simulink model "SiEngine"  (R2020a)
settings: Solver=VariableStepAuto  StartTime=0.0  StopTime=inf  RelTol=1e-3  EnableMultiTasking=on
model workspace (MAT data in the model file):
  AccPwrbp = [0 1.5]
  AccSpdbp = [300 750]
  AfrStoich = 14.6
  TimeCnstECP = 0.125
  TimeCnstEGR = 0.125
  TimeCnstETC = 0.085
  TimeCnstICP = 0.125
  TimeCnstIVL = 0.125
  TimeCnstSWVA = 0.125
  TimeCnstVCR = 0.125
  TimeCnstVGT = 0.15
  TimeCnstVIRL = 0.125
  TimeCnstWGA = 0.15
  f_twc_eff_co = [0.17 0.25 0.45 0.99 0.99 0.99 0.99]
  f_twc_eff_hc = [0.21 0.375 0.75 0.98 0.98 0.98 0.98]
  f_twc_eff_lam = [0.909090909 0.944055944 0.979020979 1 1.013986014 1.048951049 1.083916084]
  f_twc_eff_nox = [0.98 0.98 0.98 0.97 0.05 0.02 0]
libraries: autolibpowerinfoutils x1, autolibutils x1
settings Model: ModifiedByFormat=The MathWorks, Inc.  OrderedModelArguments=off  Creator=The MathWorks, Inc.  LastModifiedBy=The MathWorks, Inc.
settings SolverCC: DecoupledContinuousIntegration=on
settings DataIOCC: DSMLogging=off  ReturnWorkspaceOutputs=off
settings DebuggingCC: ModelReferenceExtraNoncontSigs=none  ArithmeticOperatorsInVariantConditions=warning
settings SFSimCC: SimUseLocalCustomCode=off  CustomCodeUndefinedFunction=UseInterfaceOnly
settings RTWCC: RTWUseLocalCustomCode=off
settings CodeAppCC: StateflowObjectComments=on
settings GRTTargetCC: TargetLangStandard=C89/C90 (ANSI)
settings ConfigComp: CovMetricSettings=dsw  CovHtmlReporting=on  CovSaveCumulativeToWorkspaceVar=on  CovSaveSingleToWorkspaceVar=on  CovShowResultsExplorer=off  CovExternalEMLEnable=off
settings SimscapeCC: SimscapeNormalizeSystem=off  SimscapeNominalValues={1, 'bar'; 1, 'cm^3/s'; 1, 'bar*kg/s'; 1, 'kJ/kg'; 1, 'kW'; };

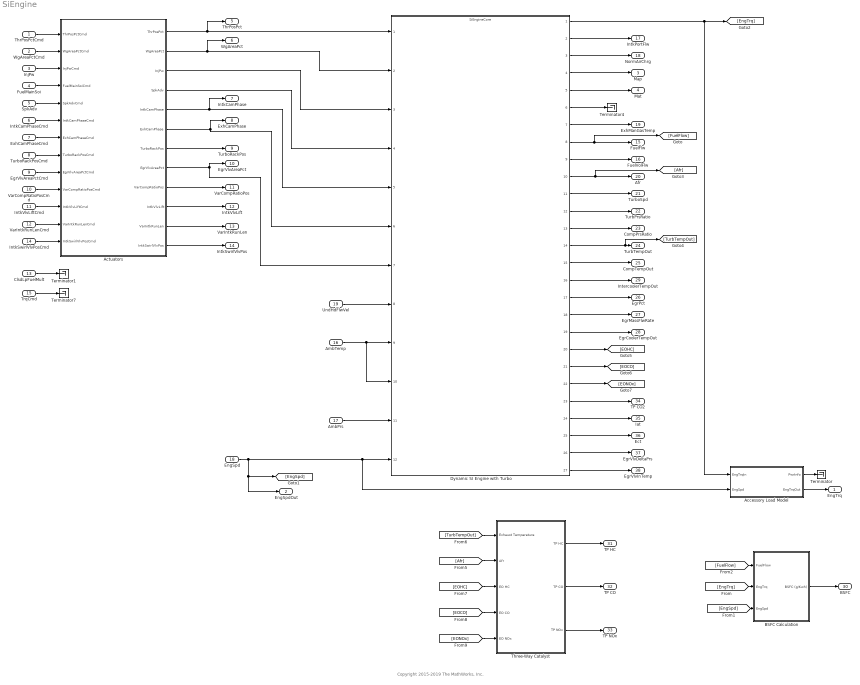
== system SiEngine ==
  note: Copyright 2015-2019 The MathWorks, Inc.
  ThrPosPctCmd : Inport
  WgAreaPctCmd : Inport  Port=2
  InjPw : Inport  Port=3
  FuelMainSoi : Inport  Port=4
  SpkAdv : Inport  Port=5
  IntkCamPhaseCmd : Inport  Port=6
  ExhCamPhaseCmd : Inport  Port=7
  TurboRackPosCmd : Inport  Port=8
  EgrVlvAreaPctCmd : Inport  Port=9
  VarCompRatioPosCmd : Inport  Port=10
  IntkVlvLiftCmd : Inport  Port=11
  VarIntkRunLenCmd : Inport  Port=12
  ClsdLpFuelMult : Inport  Port=13  Unit=1
  IntkSwirlVlvPosCmd : Inport  Port=14
  TrqCmd : Inport  Port=15  Unit=N*m
  AmbTemp : Inport  Port=16
  AmbPrs : Inport  Port=17
  EngSpd : Inport  Port=18  Interpolate=off
  UndHdFlwVel : Inport  Port=19
  Accessory Load Model : Subsystem
  Actuators : Subsystem
  BSFC Calculation : Subsystem
  Dynamic SI Engine with Turbo : ModelReference  ModelNameDialog=SiEngineCore.slx  SimulationMode=Normal  ModelReferenceVersion=1.557
  Terminator{,1,4,7} (4 alike) : Terminator
  Three-Way Catalyst : Subsystem
  EngTrq : Outport  Unit=N*m  VectorParamsAs1DForOutWhenUnconnected=off
  EngSpdOut : Outport  Port=2  VectorParamsAs1DForOutWhenUnconnected=off
  Map : Outport  Port=3  VectorParamsAs1DForOutWhenUnconnected=off
  Mat : Outport  Port=4  VectorParamsAs1DForOutWhenUnconnected=off
  ThrPosPct : Outport  Port=5  VectorParamsAs1DForOutWhenUnconnected=off
  WgAreaPct : Outport  Port=6  VectorParamsAs1DForOutWhenUnconnected=off
  IntkCamPhase : Outport  Port=7  VectorParamsAs1DForOutWhenUnconnected=off
  ExhCamPhase : Outport  Port=8  VectorParamsAs1DForOutWhenUnconnected=off
  TurboRackPos : Outport  Port=9  VectorParamsAs1DForOutWhenUnconnected=off
  EgrVlvAreaPct : Outport  Port=10  VectorParamsAs1DForOutWhenUnconnected=off
  VarCompRatioPos : Outport  Port=11  VectorParamsAs1DForOutWhenUnconnected=off
  IntkVlvLift : Outport  Port=12  VectorParamsAs1DForOutWhenUnconnected=off
  VarIntkRunLen : Outport  Port=13  VectorParamsAs1DForOutWhenUnconnected=off
  IntkSwirlVlvPos : Outport  Port=14  VectorParamsAs1DForOutWhenUnconnected=off
  FuelFlw : Outport  Port=15  VectorParamsAs1DForOutWhenUnconnected=off
  FuelVolFlw : Outport  Port=16  VectorParamsAs1DForOutWhenUnconnected=off
  IntkPortFlw : Outport  Port=17  VectorParamsAs1DForOutWhenUnconnected=off
  NormAirChrg : Outport  Port=18  VectorParamsAs1DForOutWhenUnconnected=off
  ExhManGasTemp : Outport  Port=19  VectorParamsAs1DForOutWhenUnconnected=off
  Afr : Outport  Port=20  VectorParamsAs1DForOutWhenUnconnected=off
  TurboSpd : Outport  Port=21  VectorParamsAs1DForOutWhenUnconnected=off
  TurbPrsRatio : Outport  Port=22  VectorParamsAs1DForOutWhenUnconnected=off
  CompPrsRatio : Outport  Port=23  VectorParamsAs1DForOutWhenUnconnected=off
  TurbTempOut : Outport  Port=24  VectorParamsAs1DForOutWhenUnconnected=off
  CompTempOut : Outport  Port=25  VectorParamsAs1DForOutWhenUnconnected=off
  EgrPct : Outport  Port=26  Unit=%  VectorParamsAs1DForOutWhenUnconnected=off
  EgrMassFlwRate : Outport  Port=27  Unit=kg/s  VectorParamsAs1DForOutWhenUnconnected=off
  EgrCoolerTempOut : Outport  Port=28  Unit=K  VectorParamsAs1DForOutWhenUnconnected=off
  IntercoolerTempOut : Outport  Port=29  VectorParamsAs1DForOutWhenUnconnected=off
  BSFC : Outport  Port=30  Unit=g/(kW*hr)  VectorParamsAs1DForOutWhenUnconnected=off
  TP HC : Outport  Port=31  VectorParamsAs1DForOutWhenUnconnected=off
  TP CO : Outport  Port=32  VectorParamsAs1DForOutWhenUnconnected=off
  TP NOx : Outport  Port=33  VectorParamsAs1DForOutWhenUnconnected=off
  TP CO2 : Outport  Port=34  VectorParamsAs1DForOutWhenUnconnected=off
  Iat : Outport  Port=35  VectorParamsAs1DForOutWhenUnconnected=off
  Ect : Outport  Port=36  VectorParamsAs1DForOutWhenUnconnected=off
  EgrVlvDeltaPrs : Outport  Port=37  VectorParamsAs1DForOutWhenUnconnected=off
  EgrVlvInTemp : Outport  Port=38  VectorParamsAs1DForOutWhenUnconnected=off
  wires:
  Dynamic SI Engine with Turbo/2 -> IntkPortFlw/1
  Dynamic SI Engine with Turbo/6 -> Terminator4/1
  Dynamic SI Engine with Turbo/7 -> ExhManGasTemp/1
  Dynamic SI Engine with Turbo/4 -> Map/1
  Dynamic SI Engine with Turbo/5 -> Mat/1
  SpkAdv/1 -> Actuators/5(SpkAdvCmd)
  InjPw/1 -> Actuators/3(InjPwCmd)
  EngSpd/1 -> EngSpdOut/1, [EngSpd], Dynamic SI Engine with Turbo/12, Accessory Load Model/2(EngSpd)
  [FuelFlow] -> BSFC Calculation/1(FuelFlow)
  [EngTrq] -> BSFC Calculation/2(EngTrq)
  [EngSpd] -> BSFC Calculation/3(EngSpd)
  BSFC Calculation/1(BSFC (g/Kwh)) -> BSFC/1
  Dynamic SI Engine with Turbo/1 -> Accessory Load Model/1(EngTrqIn), [EngTrq]
  Three-Way Catalyst/1(TP HC) -> TP HC/1
  Three-Way Catalyst/2(TP CO) -> TP CO/1
  Three-Way Catalyst/3(TP NOx) -> TP NOx/1
  [TurbTempOut] -> Three-Way Catalyst/1(Exhaust Temperature)
  [Afr] -> Three-Way Catalyst/2(Afr)
  ThrPosPctCmd/1 -> Actuators/1(ThrPosPctCmd)
  WgAreaPctCmd/1 -> Actuators/2(WgAreaPctCmd)
  IntkCamPhaseCmd/1 -> Actuators/6(IntkCamPhaseCmd)
  ExhCamPhaseCmd/1 -> Actuators/7(ExhCamPhaseCmd)
  Dynamic SI Engine with Turbo/8 -> [FuelFlow], FuelFlw/1
  Dynamic SI Engine with Turbo/10 -> [Afr], Afr/1
  TrqCmd/1 -> Terminator7/1
  Dynamic SI Engine with Turbo/3 -> NormAirChrg/1
  Dynamic SI Engine with Turbo/14 -> TurbTempOut/1, [TurbTempOut]
  [EOHC] -> Three-Way Catalyst/3(EO HC)
  [EOCO] -> Three-Way Catalyst/4(EO CO)
  [EONOx] -> Three-Way Catalyst/5(EO NOx)
  UndHdFlwVel/1 -> Dynamic SI Engine with Turbo/8
  AmbTemp/1 -> Dynamic SI Engine with Turbo/10, Dynamic SI Engine with Turbo/9
  AmbPrs/1 -> Dynamic SI Engine with Turbo/11
  Actuators/1(ThrPosPct) -> Dynamic SI Engine with Turbo/1, ThrPosPct/1
  Actuators/2(WgAreaPct) -> Dynamic SI Engine with Turbo/2, WgAreaPct/1
  Actuators/3(InjPw) -> Dynamic SI Engine with Turbo/3
  Actuators/4(SpkAdv) -> Dynamic SI Engine with Turbo/4
  Actuators/5(IntkCamPhase) -> Dynamic SI Engine with Turbo/5, IntkCamPhase/1
  Actuators/6(ExhCamPhase) -> Dynamic SI Engine with Turbo/6, ExhCamPhase/1
  FuelMainSoi/1 -> Actuators/4(FuelMainSoiCmd)
  TurboRackPosCmd/1 -> Actuators/8(TurboRackPosCmd)
  EgrVlvAreaPctCmd/1 -> Actuators/9(EgrVlvAreaPctCmd)
  VarCompRatioPosCmd/1 -> Actuators/10(VarCompRatioPosCmd)
  IntkVlvLiftCmd/1 -> Actuators/11(IntkVlvLiftCmd)
  VarIntkRunLenCmd/1 -> Actuators/12(VarIntkRunLenCmd)
  IntkSwirlVlvPosCmd/1 -> Actuators/13(IntkSwirlVlvPosCmd)
  Actuators/7(TurboRackPos) -> TurboRackPos/1
  Actuators/8(EgrVlvAreaPct) -> Dynamic SI Engine with Turbo/7, EgrVlvAreaPct/1
  Actuators/9(VarCompRatioPos) -> VarCompRatioPos/1
  Actuators/10(IntkVlvLift) -> IntkVlvLift/1
  Actuators/11(VarIntkRunLen) -> VarIntkRunLen/1
  Actuators/12(IntkSwirlVlvPos) -> IntkSwirlVlvPos/1
  Dynamic SI Engine with Turbo/15 -> CompTempOut/1
  Dynamic SI Engine with Turbo/16 -> IntercoolerTempOut/1
  Dynamic SI Engine with Turbo/13 -> CompPrsRatio/1
  Dynamic SI Engine with Turbo/12 -> TurbPrsRatio/1
  Dynamic SI Engine with Turbo/11 -> TurboSpd/1
  Dynamic SI Engine with Turbo/23 -> TP CO2/1
  Dynamic SI Engine with Turbo/22 -> [EONOx]
  Dynamic SI Engine with Turbo/21 -> [EOCO]
  Dynamic SI Engine with Turbo/20 -> [EOHC]
  Dynamic SI Engine with Turbo/17 -> EgrPct/1
  Dynamic SI Engine with Turbo/18 -> EgrMassFlwRate/1
  Dynamic SI Engine with Turbo/19 -> EgrCoolerTempOut/1
  Dynamic SI Engine with Turbo/25 -> Ect/1
  Dynamic SI Engine with Turbo/26 -> EgrVlvDeltaPrs/1
  Dynamic SI Engine with Turbo/27 -> EgrVlvInTemp/1
  Dynamic SI Engine with Turbo/24 -> Iat/1
  Accessory Load Model/2(EngTrqOut) -> EngTrq/1
  Accessory Load Model/1(PwrInfo) -> Terminator/1
  Dynamic SI Engine with Turbo/9 -> FuelVolFlw/1
  ClsdLpFuelMult/1 -> Terminator1/1

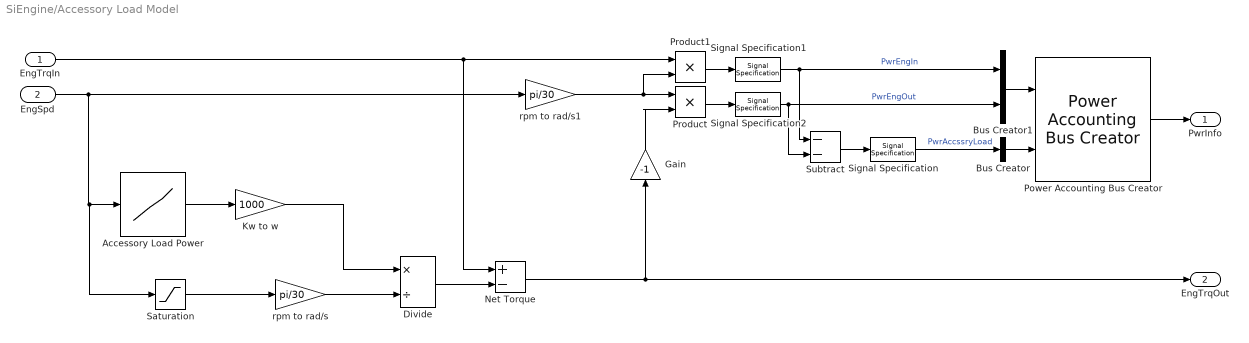
== system SiEngine/Accessory Load Model ==
  EngTrqIn : Inport
  EngSpd : Inport  Port=2
  Accessory Load Power : Lookup_n-D  NumberOfTableDimensions=1  LookupTableObject=''  BreakpointsForDimension1=AccSpdbp  Table=AccPwrbp  ExtrapMethod=Clip  InternalRulePriority=Speed  RndMeth=Simplest  InputSameDT=on
  Bus Creator : BusCreator  Inputs=1
  Bus Creator1 : BusCreator  Inputs=2
  Divide : Product  Inputs=*/
  Gain : Gain  Gain=-1
  Kw to w : Gain  Gain=1000
  Net Torque : Sum  Inputs=+-
  Power Accounting Bus Creator : autolibpowerinfoutils/Power Accounting Bus Creator  AssctBlkSelPopup=Parent  RefBlkName='libraryname/blkname'  PwrTrnsfrdCheckBox=on  PwrNotTrnsfrdCheckBox=on  PwrStoredCheckBox=off  aMode=aMode
      settings: SourceProductBaseCode=PW,MT,VE,VP
  Product : Product
  Product1 : Product
  Saturation : Saturate  UpperLimit=Inf  LowerLimit=300
  Signal Specification : SignalSpecification  Unit=W
  Signal Specification1 : SignalSpecification  Unit=W
  Signal Specification2 : SignalSpecification  Unit=W
  Subtract : Sum  Inputs=--
  rpm to rad/s : Gain  Gain=pi/30
  rpm to rad/s1 : Gain  Gain=pi/30
  PwrInfo : Outport  VectorParamsAs1DForOutWhenUnconnected=off
  EngTrqOut : Outport  Port=2  Unit=N*m  VectorParamsAs1DForOutWhenUnconnected=off
  wires:
  Divide/1 -> Net Torque/2
  Accessory Load Power/1 -> Kw to w/1
  EngSpd/1 -> Saturation/1, Accessory Load Power/1, rpm to rad/s1/1
  Saturation/1 -> rpm to rad/s/1
  rpm to rad/s/1 -> Divide/2
  Net Torque/1 -> EngTrqOut/1, Gain/1
  Bus Creator/1 -> Power Accounting Bus Creator/2
  Kw to w/1 -> Divide/1
  Bus Creator1/1 -> Power Accounting Bus Creator/1
  EngTrqIn/1 -> Product1/1, Net Torque/1
  Subtract/1 -> Signal Specification/1
  Signal Specification/1 -> Bus Creator/1  "PwrAccssryLoad"
  Power Accounting Bus Creator/1 -> PwrInfo/1
  Product/1 -> Signal Specification2/1
  Product1/1 -> Signal Specification1/1
  rpm to rad/s1/1 -> Product1/2, Product/1
  Signal Specification1/1 -> Subtract/1, Bus Creator1/1  "PwrEngIn"
  Signal Specification2/1 -> Subtract/2, Bus Creator1/2  "PwrEngOut"
  Gain/1 -> Product/2

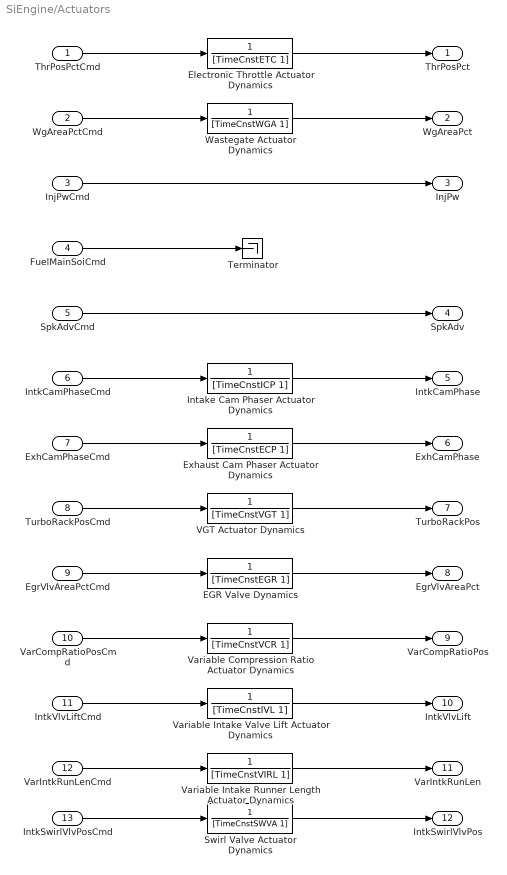
== system SiEngine/Actuators ==
  ThrPosPctCmd : Inport  Unit=%
  WgAreaPctCmd : Inport  Port=2  Unit=%
  InjPwCmd : Inport  Port=3  Unit=ms
  FuelMainSoiCmd : Inport  Port=4  Unit=deg
  SpkAdvCmd : Inport  Port=5  Unit=deg
  IntkCamPhaseCmd : Inport  Port=6  Unit=deg
  ExhCamPhaseCmd : Inport  Port=7  Unit=deg
  TurboRackPosCmd : Inport  Port=8  Unit=1
  EgrVlvAreaPctCmd : Inport  Port=9  Unit=%
  VarCompRatioPosCmd : Inport  Port=10
  IntkVlvLiftCmd : Inport  Port=11
  VarIntkRunLenCmd : Inport  Port=12
  IntkSwirlVlvPosCmd : Inport  Port=13
  EGR Valve Dynamics : TransferFcn  Denominator=[TimeCnstEGR 1]
  Electronic Throttle Actuator Dynamics : TransferFcn  Denominator=[TimeCnstETC 1]
  Exhaust Cam Phaser Actuator Dynamics : TransferFcn  Denominator=[TimeCnstECP 1]
  Intake Cam Phaser Actuator Dynamics : TransferFcn  Denominator=[TimeCnstICP 1]
  Swirl Valve Actuator Dynamics : TransferFcn  Denominator=[TimeCnstSWVA 1]
  Terminator : Terminator
  VGT Actuator Dynamics : TransferFcn  Denominator=[TimeCnstVGT 1]
  Variable Compression Ratio Actuator Dynamics : TransferFcn  Denominator=[TimeCnstVCR 1]
  Variable Intake Runner Length Actuator Dynamics : TransferFcn  Denominator=[TimeCnstVIRL 1]
  Variable Intake Valve Lift Actuator Dynamics : TransferFcn  Denominator=[TimeCnstIVL 1]
  Wastegate Actuator Dynamics : TransferFcn  Denominator=[TimeCnstWGA 1]
  ThrPosPct : Outport  Unit=%  VectorParamsAs1DForOutWhenUnconnected=off
  WgAreaPct : Outport  Port=2  Unit=%  VectorParamsAs1DForOutWhenUnconnected=off
  InjPw : Outport  Port=3  VectorParamsAs1DForOutWhenUnconnected=off
  SpkAdv : Outport  Port=4  VectorParamsAs1DForOutWhenUnconnected=off
  IntkCamPhase : Outport  Port=5  Unit=deg  VectorParamsAs1DForOutWhenUnconnected=off
  ExhCamPhase : Outport  Port=6  Unit=deg  VectorParamsAs1DForOutWhenUnconnected=off
  TurboRackPos : Outport  Port=7  Unit=1  VectorParamsAs1DForOutWhenUnconnected=off
  EgrVlvAreaPct : Outport  Port=8  Unit=%  VectorParamsAs1DForOutWhenUnconnected=off
  VarCompRatioPos : Outport  Port=9  VectorParamsAs1DForOutWhenUnconnected=off
  IntkVlvLift : Outport  Port=10  VectorParamsAs1DForOutWhenUnconnected=off
  VarIntkRunLen : Outport  Port=11  VectorParamsAs1DForOutWhenUnconnected=off
  IntkSwirlVlvPos : Outport  Port=12  VectorParamsAs1DForOutWhenUnconnected=off
  wires:
  Variable Compression Ratio Actuator Dynamics/1 -> VarCompRatioPos/1
  Variable Intake Valve Lift Actuator Dynamics/1 -> IntkVlvLift/1
  Variable Intake Runner Length Actuator Dynamics/1 -> VarIntkRunLen/1
  Swirl Valve Actuator Dynamics/1 -> IntkSwirlVlvPos/1
  Intake Cam Phaser Actuator Dynamics/1 -> IntkCamPhase/1
  Exhaust Cam Phaser Actuator Dynamics/1 -> ExhCamPhase/1
  Wastegate Actuator Dynamics/1 -> WgAreaPct/1
  Electronic Throttle Actuator Dynamics/1 -> ThrPosPct/1
  FuelMainSoiCmd/1 -> Terminator/1
  IntkVlvLiftCmd/1 -> Variable Intake Valve Lift Actuator Dynamics/1
  IntkSwirlVlvPosCmd/1 -> Swirl Valve Actuator Dynamics/1
  WgAreaPctCmd/1 -> Wastegate Actuator Dynamics/1
  ThrPosPctCmd/1 -> Electronic Throttle Actuator Dynamics/1
  ExhCamPhaseCmd/1 -> Exhaust Cam Phaser Actuator Dynamics/1
  IntkCamPhaseCmd/1 -> Intake Cam Phaser Actuator Dynamics/1
  VarCompRatioPosCmd/1 -> Variable Compression Ratio Actuator Dynamics/1
  VarIntkRunLenCmd/1 -> Variable Intake Runner Length Actuator Dynamics/1
  InjPwCmd/1 -> InjPw/1
  VGT Actuator Dynamics/1 -> TurboRackPos/1
  EGR Valve Dynamics/1 -> EgrVlvAreaPct/1
  TurboRackPosCmd/1 -> VGT Actuator Dynamics/1
  EgrVlvAreaPctCmd/1 -> EGR Valve Dynamics/1
  SpkAdvCmd/1 -> SpkAdv/1

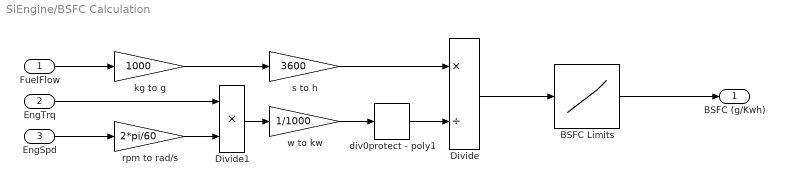
== system SiEngine/BSFC Calculation ==
  FuelFlow : Inport
  EngTrq : Inport  Port=2
  EngSpd : Inport  Port=3
  BSFC Limits : Lookup_n-D  NumberOfTableDimensions=1  BreakpointsForDimension1=[0 500]  Table=[0 500]  ExtrapMethod=Clip  InternalRulePriority=Speed  RndMeth=Simplest  InputSameDT=on
  Divide : Product  Inputs=*/
  Divide1 : Product  Inputs=**
  div0protect - poly1 : autolibutils/div0protect - poly  thresh=1e-6  aMode=aMode
      settings: SourceProductBaseCode=PW,MT,VE,VP
  kg to g : Gain  Gain=1000
  rpm to rad/s : Gain  Gain=2*pi/60
  s to h : Gain  Gain=3600
  w to kw : Gain  Gain=1/1000
  BSFC (g/Kwh) : Outport  VectorParamsAs1DForOutWhenUnconnected=off
  wires:
  Divide1/1 -> w to kw/1
  kg to g/1 -> s to h/1
  FuelFlow/1 -> kg to g/1
  rpm to rad/s/1 -> Divide1/2
  EngSpd/1 -> rpm to rad/s/1
  EngTrq/1 -> Divide1/1
  Divide/1 -> BSFC Limits/1
  w to kw/1 -> div0protect - poly1/1
  s to h/1 -> Divide/1
  BSFC Limits/1 -> BSFC (g/Kwh)/1
  div0protect - poly1/1 -> Divide/2

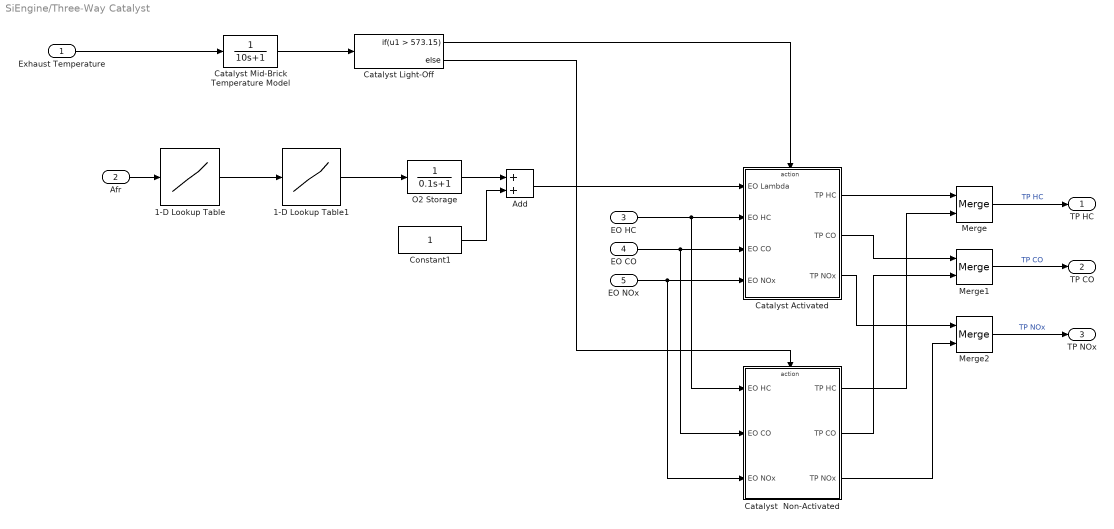
== system SiEngine/Three-Way Catalyst ==
  Exhaust Temperature : Inport
  Afr : Inport  Port=2
  EO HC : Inport  Port=3
  EO CO : Inport  Port=4
  EO NOx : Inport  Port=5
  1-D Lookup Table : Lookup_n-D  NumberOfTableDimensions=1  BreakpointsForDimension1=[0 15 100]  Table=[0 15 AfrStoich]/AfrStoich  ExtrapMethod=Clip  InternalRulePriority=Speed  RndMeth=Simplest  InputSameDT=on
  1-D Lookup Table1 : Lookup_n-D  NumberOfTableDimensions=1  BreakpointsForDimension1=[0 0.97 1.03 1.1]  Table=[-1 0 0 0.07]  ExtrapMethod=Clip  InternalRulePriority=Speed  RndMeth=Simplest  InputSameDT=on
  Add : Sum
  Catalyst  Non-Activated : Subsystem
  Catalyst Activated : Subsystem
  Catalyst Light-Off : If  IfExpression=u1 > 573.15
  "Catalyst Mid-Brick Temperature Model " : TransferFcn  Denominator=[10 1]
  Constant1 : Constant
  Merge : Merge
  Merge1 : Merge
  Merge2 : Merge
  O2 Storage : TransferFcn  Denominator=[0.1 1]
  TP HC : Outport  Unit=kg/s  VectorParamsAs1DForOutWhenUnconnected=off
  TP CO : Outport  Port=2  Unit=kg/s  VectorParamsAs1DForOutWhenUnconnected=off
  TP NOx : Outport  Port=3  Unit=kg/s  VectorParamsAs1DForOutWhenUnconnected=off
  wires:
  EO HC/1 -> Catalyst  Non-Activated/1(EO HC), Catalyst Activated/2(EO HC)
  EO CO/1 -> Catalyst  Non-Activated/2(EO CO), Catalyst Activated/3(EO CO)
  EO NOx/1 -> Catalyst  Non-Activated/3(EO NOx), Catalyst Activated/4(EO NOx)
  Merge/1 -> TP HC/1  "TP HC"
  Merge1/1 -> TP CO/1  "TP CO"
  Merge2/1 -> TP NOx/1  "TP NOx"
  Exhaust Temperature/1 -> "Catalyst Mid-Brick Temperature Model "/1
  Catalyst Light-Off/1 -> Catalyst Activated/Action
  Catalyst Light-Off/2 -> Catalyst  Non-Activated/Action
  "Catalyst Mid-Brick Temperature Model "/1 -> Catalyst Light-Off/1
  Catalyst Activated/1(TP HC) -> Merge/1
  Catalyst  Non-Activated/1(TP HC) -> Merge/2
  Catalyst Activated/2(TP CO) -> Merge1/1
  Catalyst  Non-Activated/2(TP CO) -> Merge1/2
  Catalyst Activated/3(TP NOx) -> Merge2/1
  Catalyst  Non-Activated/3(TP NOx) -> Merge2/2
  Add/1 -> Catalyst Activated/1(EO Lambda)
  1-D Lookup Table1/1 -> O2 Storage/1
  Constant1/1 -> Add/2
  O2 Storage/1 -> Add/1
  Afr/1 -> 1-D Lookup Table/1
  1-D Lookup Table/1 -> 1-D Lookup Table1/1

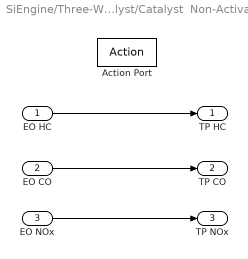
== system SiEngine/Three-Way Catalyst/Catalyst  Non-Activated ==
  EO HC : Inport
  EO CO : Inport  Port=2
  EO NOx : Inport  Port=3
  Action Port : ActionPort  ActionPortLabel=else { }
  TP HC : Outport  VectorParamsAs1DForOutWhenUnconnected=off
  TP CO : Outport  Port=2  VectorParamsAs1DForOutWhenUnconnected=off
  TP NOx : Outport  Port=3  VectorParamsAs1DForOutWhenUnconnected=off
  wires:
  EO HC/1 -> TP HC/1
  EO CO/1 -> TP CO/1
  EO NOx/1 -> TP NOx/1

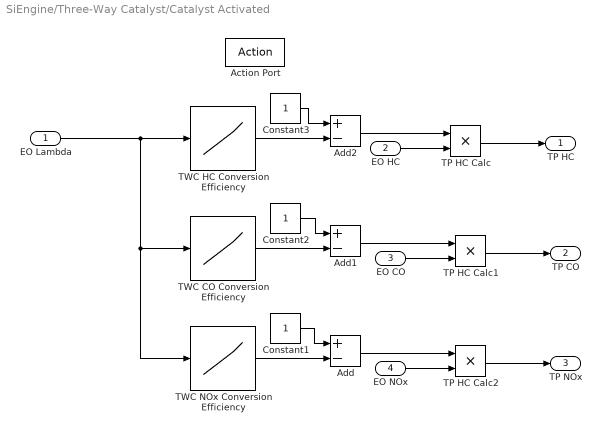
== system SiEngine/Three-Way Catalyst/Catalyst Activated ==
  EO Lambda : Inport
  EO HC : Inport  Port=2
  EO CO : Inport  Port=3
  EO NOx : Inport  Port=4
  Action Port : ActionPort  ActionPortLabel=if { }
  Add : Sum  Inputs=+-
  Add1 : Sum  Inputs=+-
  Add2 : Sum  Inputs=+-
  Constant1 : Constant
  Constant2 : Constant
  Constant3 : Constant
  TP HC Calc : Product  Inputs=**
  TP HC Calc1 : Product  Inputs=**
  TP HC Calc2 : Product  Inputs=**
  TWC CO Conversion Efficiency : Lookup_n-D  NumberOfTableDimensions=1  LookupTableObject=''  BreakpointsForDimension1=f_twc_eff_lam  Table=f_twc_eff_co  ExtrapMethod=Clip  InternalRulePriority=Speed  RndMeth=Simplest  InputSameDT=on
  TWC HC Conversion Efficiency : Lookup_n-D  NumberOfTableDimensions=1  LookupTableObject=''  BreakpointsForDimension1=f_twc_eff_lam  Table=f_twc_eff_hc  ExtrapMethod=Clip  InternalRulePriority=Speed  RndMeth=Simplest  InputSameDT=on
  TWC NOx Conversion Efficiency : Lookup_n-D  NumberOfTableDimensions=1  LookupTableObject=''  BreakpointsForDimension1=f_twc_eff_lam  Table=f_twc_eff_nox  ExtrapMethod=Clip  InternalRulePriority=Speed  RndMeth=Simplest  InputSameDT=on
  TP HC : Outport  VectorParamsAs1DForOutWhenUnconnected=off
  TP CO : Outport  Port=2  VectorParamsAs1DForOutWhenUnconnected=off
  TP NOx : Outport  Port=3  VectorParamsAs1DForOutWhenUnconnected=off
  wires:
  EO HC/1 -> TP HC Calc/2
  TP HC Calc/1 -> TP HC/1
  Add/1 -> TP HC Calc2/1
  Constant1/1 -> Add/1
  TP HC Calc1/1 -> TP CO/1
  TWC HC Conversion Efficiency/1 -> Add2/2
  Add1/1 -> TP HC Calc1/1
  EO CO/1 -> TP HC Calc1/2
  TP HC Calc2/1 -> TP NOx/1
  EO NOx/1 -> TP HC Calc2/2
  EO Lambda/1 -> TWC NOx Conversion Efficiency/1, TWC CO Conversion Efficiency/1, TWC HC Conversion Efficiency/1
  Constant2/1 -> Add1/1
  TWC CO Conversion Efficiency/1 -> Add1/2
  Constant3/1 -> Add2/1
  Add2/1 -> TP HC Calc/1
  TWC NOx Conversion Efficiency/1 -> Add/2
